simulink model "slosh_simulink_SpringMassDamper"  (R2022b)
settings: Solver=VariableStepAuto  StartTime=0.0  StopTime=20  RelTol=1e-3
values from neighbouring files (symbols this model uses):
  mVehicle = 1.6*10^4    (= 16000)    [start_slosh_state_space.m]
undefined symbols (not defined in the file or in its folder): C_0, dampingCoeffMatrix, KVehicle, massMatrix, stiffnessCoeffMatrix
settings Model: Creator=trameshk  LastModifiedBy=trameshk

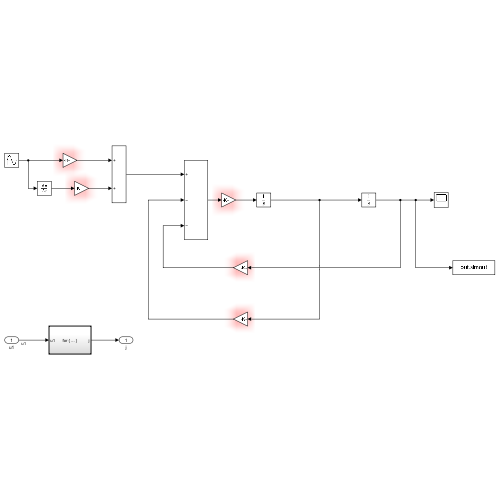
[thumbnail: Simulink's stored preview of the top-level diagram]
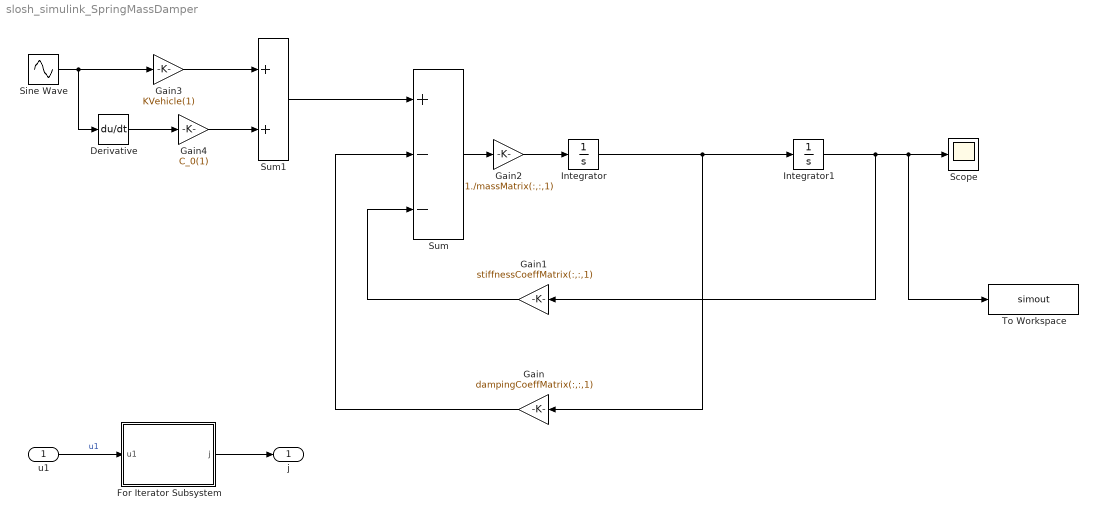
== system slosh_simulink_SpringMassDamper ==
  u1 : Inport  OutDataTypeStr=int32  PortDimensions=10
  Derivative : Derivative
  For Iterator Subsystem : Subsystem  TreatAsAtomicUnit=on
  Gain : Gain  Gain=dampingCoeffMatrix(:,:,1)
  Gain1 : Gain  Gain=stiffnessCoeffMatrix(:,:,1)
  Gain2 : Gain  Gain=1./massMatrix(:,:,1)
  Gain3 : Gain  Gain=KVehicle(1)
  Gain4 : Gain  Gain=C_0(1)
  Integrator : Integrator
  Integrator1 : Integrator
  Scope : Scope
  Sine Wave : Sin  Frequency=2*pi*1.6  SampleTime=0
  Sum : Sum  Inputs=+--
  Sum1 : Sum
  To Workspace : ToWorkspace  VariableName=simout  SaveFormat=Timeseries  SampleTime=-1
  j : Outport  VectorParamsAs1DForOutWhenUnconnected=off
  wires:
  Integrator/1 -> Gain/1, Integrator1/1
  Sum/1 -> Gain2/1
  For Iterator Subsystem/1(j) -> j/1
  u1/1 -> For Iterator Subsystem/1(u1)  "u1"
  Gain/1 -> Sum/2
  Gain1/1 -> Sum/3
  Gain2/1 -> Integrator/1
  Integrator1/1 -> Gain1/1, To Workspace/1, Scope/1
  Sine Wave/1 -> Derivative/1, Gain3/1
  Gain3/1 -> Sum1/1
  Sum1/1 -> Sum/1
  Derivative/1 -> Gain4/1
  Gain4/1 -> Sum1/2

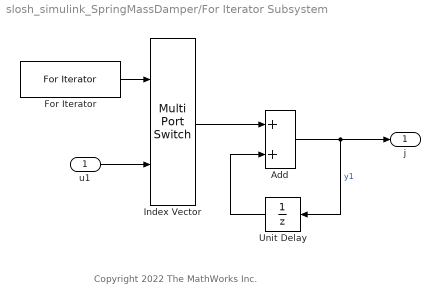
== system slosh_simulink_SpringMassDamper/For Iterator Subsystem ==
  note: Copyright 2022 The MathWorks Inc.
  u1 : Inport  OutDataTypeStr=int32
  Add : Sum
  For Iterator : ForIterator  IterationLimit=length(mVehicle)  IndexMode=Zero-based
  Index Vector : MultiPortSwitch  DataPortOrder=Zero-based contiguous  Inputs=1  zeroidx=on  SaturateOnIntegerOverflow=off  InputSameDT=off
  Unit Delay : UnitDelay  SampleTime=-1  HasFrameUpgradeWarning=on
  j : Outport  OutDataTypeStr=int32  VectorParamsAs1DForOutWhenUnconnected=off
  wires:
  u1/1 -> Index Vector/2
  For Iterator/1 -> Index Vector/1
  Index Vector/1 -> Add/1
  Unit Delay/1 -> Add/2
  Add/1 -> j/1, Unit Delay/1  "y1"
